simulink model "pendubotG_send_viet"  (R2017b)
settings: Solver=FixedStepAuto  StartTime=0.0  StopTime=10.0  FixedStep=0.01  RelTol=1e-3
values from neighbouring files (symbols this model uses):
  q1_d_init = 0.0001    [goc_init.m]
  q1_init = pi/2+0.001    (= 1.57179632679)    [goc_init.m]
  q2_d_init = 0.02    [goc_init.m]
  q2_init = 0.007    [goc_init.m]
settings Model: Creator=vohuu  LastModifiedBy=DELL
settings DebuggingCC: UnconnectedInputMsg=none  UnconnectedOutputMsg=none  UnconnectedLineMsg=none  SFMachineParentedDataDiag=error
settings SFSimCC: SimUseLocalCustomCode=on
settings RTWCC: RTWUseLocalCustomCode=on
settings CodeAppCC: StateflowObjectComments=on

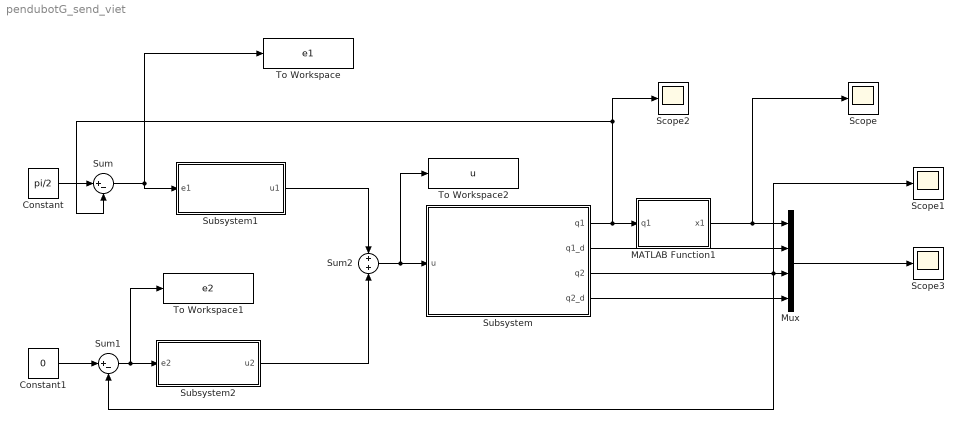
== system pendubotG_send_viet ==
  Constant : Constant  Value=pi/2
  Constant1 : Constant  Value=0
  MATLAB Function1 : MATLAB Function  TreatAsAtomicUnit=on
  Mux : Mux
  Scope{,1..3} (4 alike) : Scope
  Subsystem : Subsystem
  Subsystem1 : Subsystem
  Subsystem2 : Subsystem
  Sum : Sum  Inputs=|+-
  Sum1 : Sum  Inputs=|+-
  Sum2 : Sum
  To Workspace : ToWorkspace  VariableName=e1  SampleTime=-1
  To Workspace1 : ToWorkspace  VariableName=e2  SampleTime=-1
  To Workspace2 : ToWorkspace  VariableName=u  SampleTime=-1
  wires:
  Sum1/1 -> To Workspace1/1, Subsystem2/1(e2)
  Subsystem2/1(u2) -> Sum2/2
  Subsystem1/1(u1) -> Sum2/1
  Constant1/1 -> Sum1/1
  Sum/1 -> To Workspace/1, Subsystem1/1(e1)
  Subsystem/4(q2_d) -> Mux/4
  Mux/1 -> Scope3/1
  Sum2/1 -> To Workspace2/1, Subsystem/1(u)
  Subsystem/2(q1_d) -> Mux/2
  Constant/1 -> Sum/1
  Subsystem/3(q2) -> Sum1/2, Scope1/1, Mux/3
  MATLAB Function1/1(x1) -> Scope/1, Mux/1
  Subsystem/1(q1) -> Sum/2, Scope2/1, MATLAB Function1/1(q1)

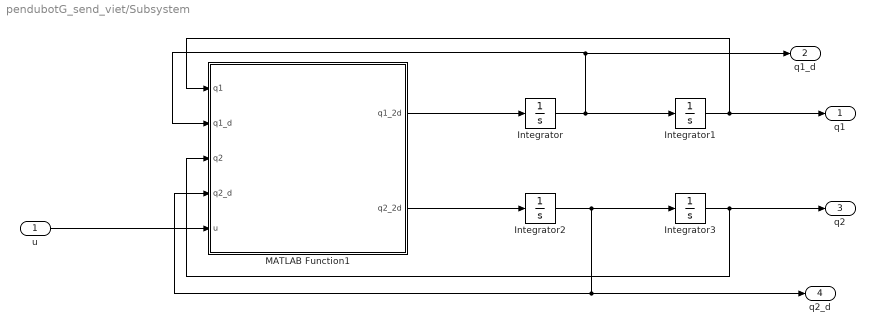
== system pendubotG_send_viet/Subsystem ==
  u : Inport
  Integrator : Integrator  InitialCondition=q1_d_init
  Integrator1 : Integrator  InitialCondition=q1_init
  Integrator2 : Integrator  InitialCondition=q2_d_init
  Integrator3 : Integrator  InitialCondition=q2_init
  MATLAB Function1 : MATLAB Function  TreatAsAtomicUnit=on
  q1 : Outport
  q1_d : Outport  Port=2
  q2 : Outport  Port=3
  q2_d : Outport  Port=4
  wires:
  Integrator2/1 -> q2_d/1, MATLAB Function1/4(q2_d), Integrator3/1
  Integrator3/1 -> MATLAB Function1/3(q2), q2/1
  Integrator/1 -> MATLAB Function1/2(q1_d), q1_d/1, Integrator1/1
  u/1 -> MATLAB Function1/5(u)
  MATLAB Function1/2(q2_2d) -> Integrator2/1
  Integrator1/1 -> MATLAB Function1/1(q1), q1/1
  MATLAB Function1/1(q1_2d) -> Integrator/1

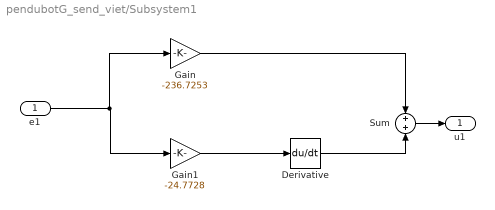
== system pendubotG_send_viet/Subsystem1 ==
  e1 : Inport
  Derivative : Derivative
  Gain : Gain  Gain=-236.7253
  Gain1 : Gain  Gain=-24.7728
  Sum : Sum
  u1 : Outport
  wires:
  Gain1/1 -> Derivative/1
  e1/1 -> Gain/1, Gain1/1
  Gain/1 -> Sum/1
  Derivative/1 -> Sum/2
  Sum/1 -> u1/1

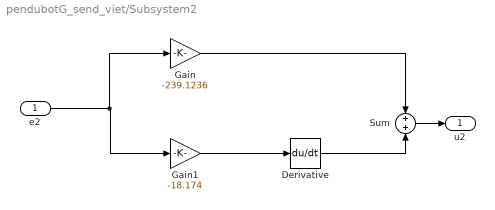
== system pendubotG_send_viet/Subsystem2 ==
  e2 : Inport
  Derivative : Derivative
  Gain : Gain  Gain=-239.1236
  Gain1 : Gain  Gain=-18.174
  Sum : Sum
  u2 : Outport
  wires:
  Derivative/1 -> Sum/2
  Gain/1 -> Sum/1
  e2/1 -> Gain/1, Gain1/1
  Sum/1 -> u2/1
  Gain1/1 -> Derivative/1

== matlab function pendubotG_send_viet/Subsystem/MATLAB Function1 ==
  data: q1 input; q1_2d output; q1_d input; q2 input; q2_d input; u input; q2_2d output
function [q1_2d,q2_2d] = fcn(q1,q1_d,q2,q2_d,u)
m1=1.068;
m2=0.07;
l1=0.146;
l2=0.253;
lc1=0.055;
lc2=0.149;
I1=0.0189;
I2=0.000409;
Kb=0.0864;
Kt=0.0864;
Rm=3.7;
Cm=0.000415;
Jm=0.000427;
g=9.80665;
K1=Kt/Rm;
K2=((Kt*Kb)/Rm)+Cm;
K3=Jm;
beta1=m1*lc1^2+m2*l1^2+I1;
beta2=m2*lc2^2+I2;
beta3=m2*l1*lc2;
beta4=m1*lc1+m2*l1;
beta5=m2*lc2;
q1_2d=1/(beta1*beta2-beta3^2*(cos(q2))^2+K3*beta2)*(beta2*beta3*sin(q2)*(q1_d+q2_d)^2+beta3^2*cos(q2)*sin(q2)*q1_d^2-beta2*beta4*g*cos(q1)+beta3*beta5*g*cos(q2)*cos(q1+q2)+beta2*K1*u-K2*beta2*q1_d);
%q2_2d=-(2*beta3^2*q1_d^2*sin(2*q2) + beta3^2*q2_d^2*sin(2*q2) - 2*K2*beta2*q1_d + 2*K1*beta2*u + 2*K3*beta5*g*cos(q1 + q2) + 2*beta1*beta5*g*cos(q1 + q2) - beta3*beta4*g*cos(q1 + q2) + 2*beta3^2*q1_d*q2_d*sin(2*q2) - 2*K2*beta3*q1_d*cos(q2) + 2*K1*beta3*u*cos(q2) - 2*beta2*beta4*g*cos(q1) + beta3*beta5*g*cos(q1) - beta3*beta4*g*cos(q1 - q2) + beta3*beta5*g*cos(q1 + 2*q2) + 2*K3*beta3*q1_d^2*sin(q2) + 2*beta1*beta3*q1_d^2*sin(q2) + 2*beta2*beta3*q1_d^2*sin(q2) + 2*beta2*beta3*q2_d^2*sin(q2) + 4*beta2*beta3*q1_d*q2_d*sin(q2))/(2*K3*beta2 + 2*beta1*beta2 - beta3^2*cos(2*q2) - beta3^2);
q2_2d=-(beta5*g*cos(q1 + q2)*(K3 + beta1 + beta3*cos(q2)) - beta4*g*cos(q1)*(beta2 + beta3*cos(q2)) - K2*q1_d*(beta2 + beta3*cos(q2)) + beta3*sin(q2)*(q1_d + q2_d)^2*(beta2 + beta3*cos(q2)) + K3*beta3*q1_d^2*sin(q2) + beta3*q1_d^2*sin(q2)*(beta1 + beta3*cos(q2)))/(- beta3^2*cos(q2)^2 + K3*beta2 + beta1*beta2) - (K1*u*(beta2 + beta3*cos(q2)))/(- beta3^2*cos(q2)^2 + K3*beta2 + beta1*beta2);

== matlab function pendubotG_send_viet/MATLAB Function1 ==
  data: q1 input; x1 output
function x1 = fcn(q1)

x1 = q1-pi/2;
